simulink model "model_backward"  (R2022a)
settings: Solver=FixedStepDiscrete  StartTime=0.0  StopTime=inf  FixedStep=5e-3  RelTol=1e-3
values from neighbouring files (symbols this model uses):
  emin = 0.1    [simulate.m]
  gamma = 0.3    [simulate.m]
  k = 1    [simulate.m]
  omega_max = (pi/180)*300    (= 5.23598775598)    [simulate.m]
  u_max = 1.2    [simulate.m]
libraries: fuzblock x4, simulink x1
settings Model: Creator=mateu  LastModifiedBy=mateu
settings SolverCC: AlgebraicLoopSolver=TrustRegion
settings RTWCC: DLArmComputeVersion=19.05

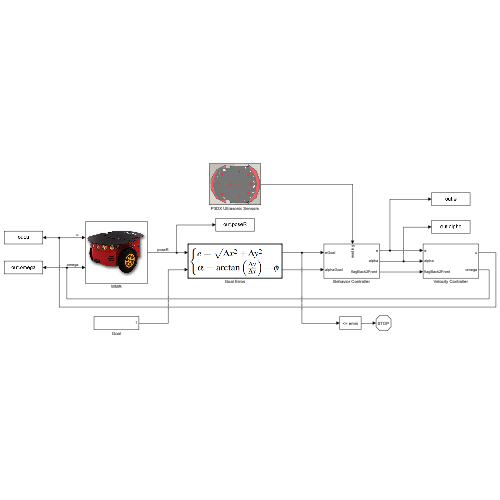
[thumbnail: Simulink's stored preview of the top-level diagram]
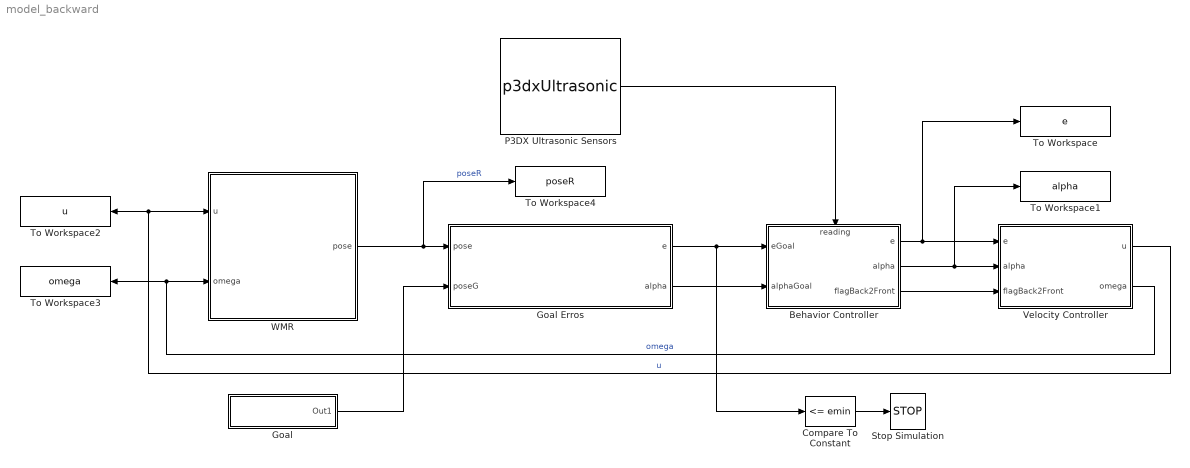
== system model_backward ==
  Behavior Controller : Subsystem
      settings: PortSchema="{\"entries\":[{\"content\":{\"sides\":[{\"content\":{\"connectorIds\":[\"In1\",\"In2\"]},\"type\":\"ConnectorPlacement.EquallySpacedRectSide\",\"uuid\":\"2b04f9f6-92c1-4971-8aaf-4a0e0d05bcd4\"},{\"content\":{\"connectorIds\":[\"Out1\",\"Out2\",\"Out3\"],\"side\":\"RIGHT\"},\"type\":\"ConnectorPlacement.EquallySpacedRectSide\",\"uuid\":\"babf92a9-9b5c-43ab-9998-a7dc1f2d324f\"},{\"content\":{\"connectorIds\":[\"In3\"],\"side\":\"TOP\"},\"type\":\"ConnectorPlacement.EquallySpacedRectSide\",\"uuid\":\"0a0c3082-370a-434d-b7bc-d0d94bfff92e\"}]},\"type\":\"ConnectorPlacement.EquallySpacedConnector\",\"uuid\":\"d36aa3a4-47e6-4710-9403-217c0656c9d5\"}],\"packageUris\":[\"http://schema.mathworks.com/mf0/Connector/R2020b\"],\"version\":\"1.0\"}"
  Compare To Constant : simulink/Logic and Bit Operations/Compare To Constant  relop=<=  const=emin  OutDataTypeStr=boolean
  Goal : Subsystem  VariantControl=GOAL_COPPELIA
  Goal Erros : MATLAB Function  TreatAsAtomicUnit=on
  P3DX Ultrasonic Sensors : M-S-Function  FunctionName=p3dxUltrasonic
      mask Display: image('$imagefile'); % Use "Edit Image" on toolstrip to change.
  Stop Simulation : Stop
  To Workspace : ToWorkspace  VariableName=e  SaveFormat=Timeseries  SampleTime=-1
  To Workspace1 : ToWorkspace  VariableName=alpha  SaveFormat=Timeseries  SampleTime=-1
  To Workspace2 : ToWorkspace  VariableName=u  SaveFormat=Timeseries  SampleTime=-1
  To Workspace3 : ToWorkspace  VariableName=omega  SaveFormat=Timeseries  SampleTime=-1
  To Workspace4 : ToWorkspace  VariableName=poseR  SaveFormat=Timeseries  SampleTime=-1
  Velocity Controller : Subsystem
  WMR : Subsystem  VariantControl=UNICYCLE_COPPELIA
      mask Display: image('$imagefile'); % Use "Edit Image" on toolstrip to change.
  wires:
  WMR/1(pose) -> To Workspace4/1, Goal Erros/1(pose)  "poseR"
  Goal/1(Out1) -> Goal Erros/2(poseG)
  Compare To Constant/1 -> Stop Simulation/1
  Velocity Controller/1(u) -> WMR/1(u), To Workspace2/1  "u"
  Velocity Controller/2(omega) -> WMR/2(omega), To Workspace3/1  "omega"
  Goal Erros/1(e) -> Behavior Controller/1(eGoal), Compare To Constant/1
  Goal Erros/2(alpha) -> Behavior Controller/2(alphaGoal)
  Behavior Controller/1(e) -> To Workspace/1, Velocity Controller/1(e)
  Behavior Controller/2(alpha) -> To Workspace1/1, Velocity Controller/2(alpha)
  Behavior Controller/3("flagBack2Front ") -> Velocity Controller/3("flagBack2Front ")
  P3DX Ultrasonic Sensors/1 -> Behavior Controller/3(reading)

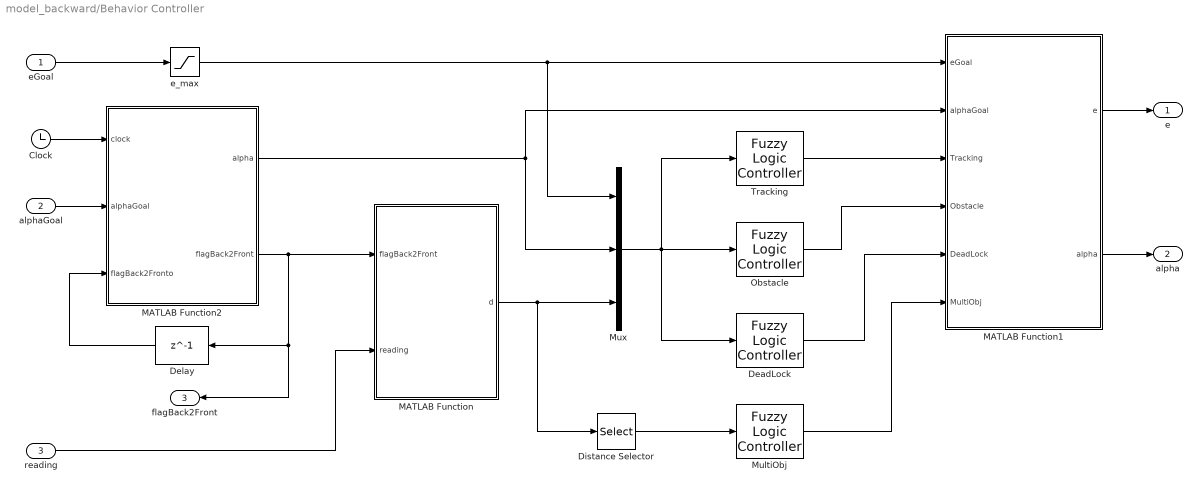
== system model_backward/Behavior Controller ==
  eGoal : Inport
  alphaGoal : Inport  Port=2
  reading : Inport  Port=3
  Clock : Clock
  DeadLock : fuzblock/Fuzzy Logic  Controller  FIS=DeadLock  OutputSampleNumber=101  DataType=double  FuzzifiedInputs=off  RuleFiringStrengths=off  RuleOutputs=off  AggregatedOutputs=off  SimulateUsing=Interpreted execution  OutOfRangeInputValueMessage=warning  NoRuleFiredMessage=warning  EmptyOutputFuzzySetMessage=warning
  Delay : Delay  DelayLength=1  InputProcessing=Columns as channels (frame based)
  Distance Selector : Selector  IndexOptions=Index vector (dialog)  Indices=[1 3 7 2 8]  OutputSizes=1
  MATLAB Function : MATLAB Function  TreatAsAtomicUnit=on
  MATLAB Function1 : MATLAB Function  TreatAsAtomicUnit=on
  MATLAB Function2 : MATLAB Function  TreatAsAtomicUnit=on
  MultiObj : fuzblock/Fuzzy Logic  Controller  FIS=Fuzzy_Behavior  OutputSampleNumber=101  DataType=double  FuzzifiedInputs=off  RuleFiringStrengths=off  RuleOutputs=off  AggregatedOutputs=off  SimulateUsing=Interpreted execution  OutOfRangeInputValueMessage=warning  NoRuleFiredMessage=warning  EmptyOutputFuzzySetMessage=warning
  Mux : Mux  Inputs=3
  "Obstacle " : fuzblock/Fuzzy Logic  Controller  FIS=Obstacle  OutputSampleNumber=101  DataType=double  FuzzifiedInputs=off  RuleFiringStrengths=off  RuleOutputs=off  AggregatedOutputs=off  SimulateUsing=Interpreted execution  OutOfRangeInputValueMessage=warning  NoRuleFiredMessage=warning  EmptyOutputFuzzySetMessage=warning
  Tracking : fuzblock/Fuzzy Logic  Controller  FIS=Tracking  OutputSampleNumber=101  DataType=double  FuzzifiedInputs=off  RuleFiringStrengths=off  RuleOutputs=off  AggregatedOutputs=off  SimulateUsing=Interpreted execution  OutOfRangeInputValueMessage=warning  NoRuleFiredMessage=warning  EmptyOutputFuzzySetMessage=warning
  e_max : Saturate  UpperLimit=3  LowerLimit=0
  e : Outport
  alpha : Outport  Port=2
  "flagBack2Front " : Outport  Port=3
  wires:
  Clock/1 -> MATLAB Function2/1(clock)
  MultiObj/1 -> MATLAB Function1/6(MultiObj)
  MATLAB Function1/1(e) -> e/1
  DeadLock/1 -> MATLAB Function1/5(DeadLock)
  Delay/1 -> MATLAB Function2/3(flagBack2Fronto)
  alphaGoal/1 -> MATLAB Function2/2(alphaGoal)
  reading/1 -> MATLAB Function/2(reading)
  e_max/1 -> Mux/1, MATLAB Function1/1(eGoal)
  MATLAB Function2/2(flagBack2Front) -> "flagBack2Front "/1, Delay/1, MATLAB Function/1(flagBack2Front)
  "Obstacle "/1 -> MATLAB Function1/4(Obstacle)
  MATLAB Function1/2(alpha) -> alpha/1
  Tracking/1 -> MATLAB Function1/3(Tracking)
  eGoal/1 -> e_max/1
  MATLAB Function2/1(alpha) -> Mux/2, MATLAB Function1/2(alphaGoal)
  MATLAB Function/1(d) -> Distance Selector/1, Mux/3
  Mux/1 -> Tracking/1, DeadLock/1, "Obstacle "/1
  Distance Selector/1 -> MultiObj/1

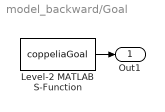
== system model_backward/Goal ==
  Level-2 MATLAB S-Function : M-S-Function  FunctionName=coppeliaGoal
  Out1 : Outport
  wires:
  Level-2 MATLAB S-Function/1 -> Out1/1

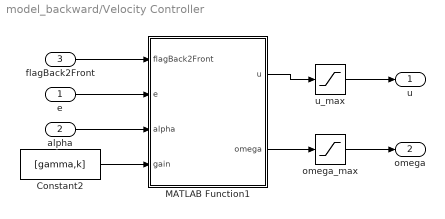
== system model_backward/Velocity Controller ==
  e : Inport
  alpha : Inport  Port=2
  "flagBack2Front " : Inport  Port=3
  Constant2 : Constant  Value=[gamma,k]
  MATLAB Function1 : MATLAB Function  TreatAsAtomicUnit=on
  omega_max : Saturate  UpperLimit=omega_max  LowerLimit=-omega_max
  u_max : Saturate  UpperLimit=u_max  LowerLimit=-u_max
  u : Outport
  omega : Outport  Port=2
  wires:
  Constant2/1 -> MATLAB Function1/4(gain)
  omega_max/1 -> omega/1
  u_max/1 -> u/1
  alpha/1 -> MATLAB Function1/3(alpha)
  e/1 -> MATLAB Function1/2(e)
  MATLAB Function1/2(omega) -> omega_max/1
  MATLAB Function1/1(u) -> u_max/1
  "flagBack2Front "/1 -> MATLAB Function1/1(flagBack2Front)

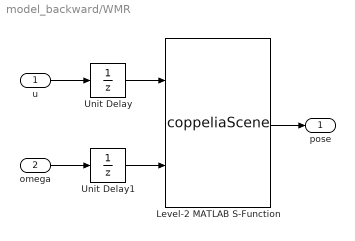
== system model_backward/WMR ==
  u : Inport
  omega : Inport  Port=2
  Level-2 MATLAB S-Function : M-S-Function  FunctionName=coppeliaScene
  Unit Delay : UnitDelay  SampleTime=-1  HasFrameUpgradeWarning=on
  Unit Delay1 : UnitDelay  SampleTime=-1  HasFrameUpgradeWarning=on
  pose : Outport
  wires:
  u/1 -> Unit Delay/1
  omega/1 -> Unit Delay1/1
  Level-2 MATLAB S-Function/1 -> pose/1
  Unit Delay/1 -> Level-2 MATLAB S-Function/1
  Unit Delay1/1 -> Level-2 MATLAB S-Function/2

== matlab function model_backward/Behavior Controller/MATLAB Function ==
  data: flagBack2Front input; reading input; d output
function d = getDistances(flagBack2Front,reading)

    
if(flagBack2Front)
    dNO = min(reading(12:13));
    dSO = min(reading(4:5));
    dES = min([reading(1),reading(16)]);
    dWE = min(reading(8:9));
    dSE = min(reading(2:3));
    dNW = min(reading(10:11));
    dNE = min(reading(14:15)); 
    dSW = min(reading(6:7));
else
    dNO = min(reading(4:5));
    dSO = min(reading(12:13));
    dES = min(reading(8:9));
    dWE = min([reading(1),reading(16)]);
    dSE = min(reading(10:11));
    dNW = min(reading(2:3));
    dNE = min(reading(6:7));
    dSW = min(reading(14:15));
end

d = [dNO,dNE,dES,dSE,dSO,dSW,dWE,dNW];

end

== matlab function model_backward/Goal Erros ==
  settings: updateMethod=DISCRETE  sampleTime=0.05
  data: pose input; e output; poseG input; alpha output
function [e,alpha] = errors(pose,poseG)

deltaX = poseG(1)-pose(1); deltaY = poseG(2)-pose(2);
phi = pose(3);

e = sqrt(deltaX^2 + deltaY^2);
alpha = atan2(deltaY,deltaX) - phi;

if alpha < -pi
    alpha = alpha + 2*pi;
elseif alpha >= pi
    alpha = alpha - 2*pi;
end

== matlab function model_backward/Velocity Controller/MATLAB Function1 ==
  settings: updateMethod=DISCRETE  sampleTime=0.05
  data: flagBack2Front input; e input; u output; alpha input; omega output; gain input
function [u,omega] = control(flagBack2Front,e,alpha,gain)

gamma = gain(1); k = gain(2);

u = gamma*e*abs(cos(alpha));
omega = k*alpha + gamma*cos(alpha)*sin(alpha);

if(flagBack2Front)
    u = -u;
end

== matlab function model_backward/Behavior Controller/MATLAB Function1 ==
  data: eGoal input; alphaGoal input; Tracking input; Obstacle input; DeadLock input; MultiObj input; e output; alpha output
function [e, alpha]  = alterStates(eGoal,alphaGoal,Tracking, Obstacle, DeadLock, MultiObj)
       
e = MultiObj(1)*eGoal+MultiObj(2)*Tracking(1)+MultiObj(3)*Obstacle(1)+MultiObj(4)*DeadLock(1);
alpha = MultiObj(1)*alphaGoal+MultiObj(2)*Tracking(2)+MultiObj(3)*Obstacle(2)+MultiObj(4)*DeadLock(2);
%     e = 2*e;
    MultiObj
  
end

== matlab function model_backward/Behavior Controller/MATLAB Function2 ==
  data: clock input; alphaGoal input; alpha output; flagBack2Front output; flagBack2Fronto input
function [alpha,flagBack2Front] = flagBack2Front(clock,alphaGoal,flagBack2Fronto)

if(clock == 0)
    alphaGoalnorm = abs(rad2deg(alphaGoal));
    flagBack2Front = double(alphaGoalnorm > 90);
else
    flagBack2Front = flagBack2Fronto;
end

if(alphaGoal > 0 && flagBack2Front)
    alpha=alphaGoal-pi;
elseif (alphaGoal < 0 && flagBack2Front)
    alpha=alphaGoal+pi;
else
    alpha=alphaGoal;
end
